simulink model "Lab3"  (Simulink 10.1)
settings: Solver=ode45  StartTime=0.0  StopTime=10.0  RelTol=1e-3  AbsTol=1e-6
libraries: dsparch4 x1
settings Model: Creator=vise  LastModifiedBy=23919  ExtModeTrigMode=oneshot  ExtModeArmWhenConnect=off
settings SolverCC: AutoScaleAbsTol=off
settings DataIOCC: SignalLoggingSaveFormat=ModelDataLogs
settings OptimizationCC: BlockReduction=off  BooleanDataType=off  ExpressionDepthLimit=2147483647  InitFltsAndDblsToZero=on
settings DebuggingCC: SaveWithParameterizedLinksMsg=none  SignalResolutionControl=TryResolveAllWithWarning  MultiTaskDSMMsg=warning  MultiTaskCondExecSysMsg=none  FcnCallInpInsideContextMsg=warning  StateNameClashWarn=warning
settings HardwareCC: TargetUnknown=on
settings RTWCC: TemplateMakefile=grt_unix.tmf

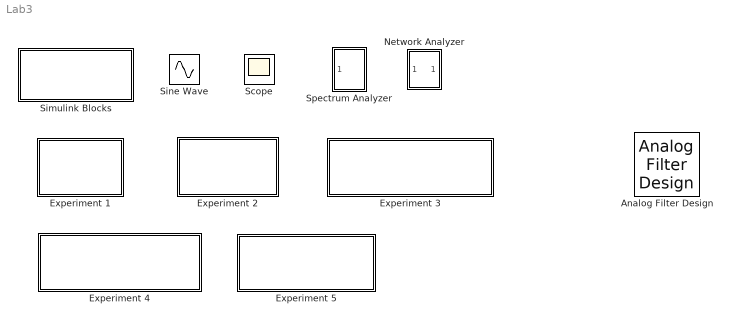
== system Lab3 ==
  Analog Filter Design : dsparch4/Analog Filter Design  method=Butterworth  filttype=Lowpass  N=8  Wlo=30  Whi=80  Rp=2  Rs=40
  Experiment 1 : Subsystem  mask(Waveform Synthesizer){}
      settings: OpenFcn=lab3Synth
      mask Display: disp('Synthesizer')
  Experiment 2 : Subsystem  mask(Modulator){}
      settings: OpenFcn=lab3Mod
      mask Display: disp('Modulator')
  Experiment 3 : Subsystem  mask(CT System Analysis/Network Analyzer){}
      settings: OpenFcn=lab3CTSys1
      mask Display: disp('CT System Analysis using\n a Network Analyzer')
  Experiment 4 : Subsystem  mask(CT System Analysis/Unit Step){}
      settings: OpenFcn=lab3CTSys2
      mask Display: disp('CT System Analysis using\n a Unit Step')
  Experiment 5 : Subsystem  mask(DT System Analysis){}
      settings: OpenFcn=lab3DTSys
      mask Display: disp('DT System Analysis')
  Network Analyzer : Subsystem  mask(Network Analyzer){Parameter1=256, Parameter2=0.1}
      mask prompts: Parameter1 "Number of sample points:"; Parameter2 "Sampling period (sec):"
      mask init:
      | max_freq=0.9*pi/@2;N=@1;T_s=@2;const=2*pi/(@1*@2);window1=0.5*@1*@2;window2=@1*@2;
      mask Help: Estimates frequency response of system using chirp input. Used for EE438. See Prof. Bouman.
      mask Display: plot(0,0,100,100,[11,93,93,11,11],[90,90,40,40,90],[80,60,40,20],[50,79,50,80])
  Scope : Scope
  Simulink Blocks : Subsystem  mask(Waveform Synthesizer){}
      settings: OpenFcn=simulink
      mask Display: disp('Full Block Library')
  Sine Wave : Sin  SampleTime=0
  Spectrum Analyzer : Subsystem  mask(Spectrum analyzer.){N=2048, T_s=0.02, plot_period=10}
      mask prompts: N "Number of sample points:"; T_s "Sampling period (sec):"; plot_period "Plotting Period (sec):"
      mask Help: EE438 Lab utility; See Prof. Bouman.
      mask Display: plot(0,0,100,100,[14,91,91,14,14],[86,86,40,40,86],[85,82,80,79,75,67,63,60,57,53,41,36,33,27,24],[49,50,53,50,49,51,54,66,54,50,50,52,81,51,49])

== system Lab3/Experiment 1 ==

== system Lab3/Experiment 2 ==

== system Lab3/Experiment 3 ==

== system Lab3/Experiment 4 ==

== system Lab3/Experiment 5 ==

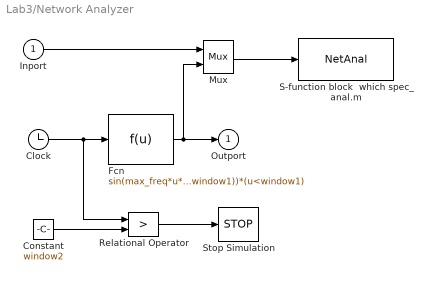
== system Lab3/Network Analyzer ==
  Inport : Inport
  Clock : Clock
  Constant : Constant  Value=window2
  Fcn : Fcn  Expr=sin(max_freq*u*u/(2*window1))*(0.54+0.46*cos(pi*u/window1))*(u<window1)
  Mux : Mux  Inputs=2
  Relational Operator : RelationalOperator  Operator=>  RndMeth=Nearest  InputSameDT=on
  S-function block  which spec_anal.m : S-Function  FunctionName=NetAnal  Parameters=N,T_s  SFunctionDeploymentMode=off  EnableBusSupport=off
  Stop Simulation : Stop
  Outport : Outport  InitialOutput=0  VectorParamsAs1DForOutWhenUnconnected=off
  wires:
  Inport/1 -> Mux/1
  Fcn/1 -> Mux/2, Outport/1
  Mux/1 -> S-function block  which spec_anal.m/1
  Clock/1 -> Fcn/1, Relational Operator/1
  Constant/1 -> Relational Operator/2
  Relational Operator/1 -> Stop Simulation/1

== system Lab3/Simulink Blocks ==

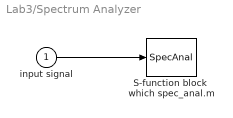
== system Lab3/Spectrum Analyzer ==
  input signal : Inport
  S-function block  which spec_anal.m : S-Function  FunctionName=SpecAnal  Parameters=N,T_s,plot_period  SFunctionDeploymentMode=off  EnableBusSupport=off
  wires:
  input signal/1 -> S-function block  which spec_anal.m/1
